simulink model "LPVmodel_Wu96_mdl"  (R2018b)
settings: Solver=ode15s  StartTime=0.0  StopTime=4  MaxStep=0.01  RelTol=1e-5  EnableMultiTasking=on
libraries: lpvlibrary x2, simulink x1
settings Model: Creator=Fernando  LastModifiedBy=ferna
settings OptimizationCC: LifeSpan=inf
settings DebuggingCC: SFUnexpectedBacktrackingDiag=warning  SFNoUnconditionalDefaultTransitionDiag=warning
settings SFSimCC: SimUseLocalCustomCode=off
settings RTWCC: RTWUseLocalCustomCode=off
settings CodeAppCC: StateflowObjectComments=on
settings GRTTargetCC: TargetLangStandard=C89/C90 (ANSI)  GeneratePreprocessorConditionals=Disable all
settings ConfigComp: CovMetricSettings=dw  CovHtmlReporting=on  CovSaveCumulativeToWorkspaceVar=on  CovSaveSingleToWorkspaceVar=on  CovExternalEMLEnable=off

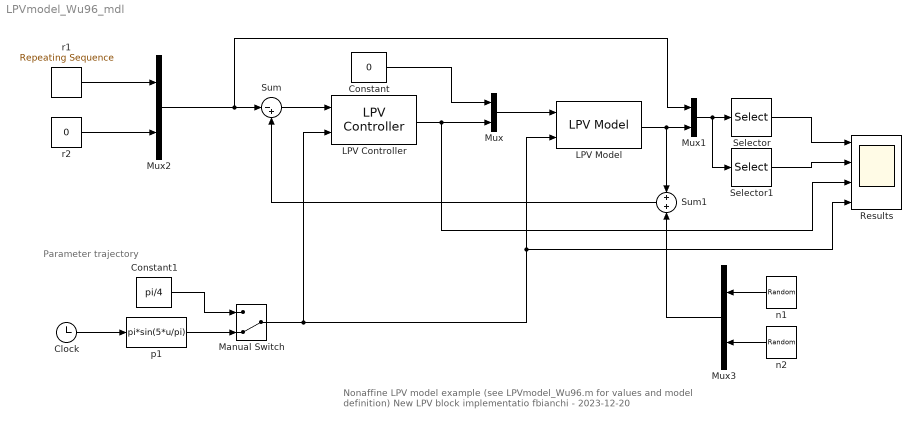
== system LPVmodel_Wu96_mdl ==
  note: Parameter trajectory
  note: Nonaffine LPV model example
      | (see LPVmodel_Wu96.m for values and model definition)
      | New LPV block implementatio
      | fbianchi - 2023-12-20
  Clock : Clock
  Constant : Constant  Value=0
  Constant1 : Constant  Value=pi/4
  LPV Controller : lpvlibrary/LPV Controller  pdK=pdK4  x0=0
      settings: SourceProductName=LPV Toolbox
  LPV Model : lpvlibrary/LPV Model  pdG=pdG  x0=0
      settings: SourceProductName=LPV Toolbox
  Manual Switch : ManualSwitch  CurrentSetting=0
  Mux : Mux  Inputs=[1 2]
  Mux1 : Mux  Inputs=[2 2]
  Mux2 : Mux  Inputs=2
  Mux3 : Mux  Inputs=2
  Results : Scope  NumInputPorts=4
  Selector : Selector  InputPortWidth=4  IndexOptions=Index vector (dialog)  Indices=[1 3]  OutputSizes=1
  Selector1 : Selector  InputPortWidth=4  IndexOptions=Index vector (dialog)  Indices=[2 4]  OutputSizes=1
  Sum : Sum  Inputs=|-+
  Sum1 : Sum
  n1 : UniformRandomNumber  Minimum=-0.005  Maximum=0.005  SampleTime=0.1
  n2 : UniformRandomNumber  Minimum=-0.005  Maximum=0.005  Seed=5565  SampleTime=0.1
  p1 : Fcn  Expr=pi*sin(5*u/pi)
  r1 : simulink/Sources/Repeating Sequence  rep_seq_t=[0 1 2 3 10]  rep_seq_y=[0 1 1 -1 -1]
  r2 : Constant  Value=0
  wires:
  Sum/1 -> LPV Controller/1
  LPV Model/1 -> Mux1/2, Sum1/1
  Mux/1 -> LPV Model/1
  Mux2/1 -> Mux1/1, Sum/1
  LPV Controller/1 -> Results/3, Mux/2
  Constant/1 -> Mux/1
  Mux1/1 -> Selector1/1, Selector/1
  Selector/1 -> Results/1
  Selector1/1 -> Results/2
  Clock/1 -> p1/1
  Constant1/1 -> Manual Switch/1
  p1/1 -> Manual Switch/2
  r1/1 -> Mux2/1
  r2/1 -> Mux2/2
  Sum1/1 -> Sum/2
  n1/1 -> Mux3/1
  n2/1 -> Mux3/2
  Mux3/1 -> Sum1/2
  Manual Switch/1 -> LPV Controller/2, LPV Model/2, Results/4
